simulink model "TSR_Scenario_002_cs"  (R2014b)
settings: Solver=ode5  SolverMode=SingleTasking  StartTime=0.0  StopTime=inf  FixedStep=1/100  RelTol=1e-3
PreLoadFcn:
  | mbxruntime.callbacks.PreLoadFcn(bdroot);
  | check_NUTS_defined;
  | 
  | assignin('base',['model_closed_' bdroot],false);
  | 
  | addpath('../includes_TSR/includes_TSR');
  | 
  | switch version('-release')
  | case {'2010a', '2010b', '2011a'}
  | addpath('../includes_TSR/ML2010b');
  | otherwise
  | addpath('../includes_TSR/ML2011b');
  | end
PostLoadFcn:
  | mbxruntime.callbacks.PostLoadFcn(bdroot);
InitFcn:
  | mbxruntime.callbacks.InitFcn(bdroot);;
  | 
  | addpath('..\includes_TSR');
StartFcn:
  | mbxruntime.callbacks.StartFcn(bdroot);
StopFcn:
  | mbxruntime.callbacks.StopFcn(bdroot);
model workspace: external: MAT-File .\TSR_Scenario_002_cs_hws.mat (data not in the file)
undefined symbols (not defined in the file or in its folder): InitImageOutputDir, mbxruntime, OrientationPitch, OrientationRoll, PositionX, PositionY, PositionZ, tabledata, warningInitialVelocity, x0
undefined symbols (not defined in the file): SteeringColumn, SteeringWheel, TSR_Scenario_002_cs_003e47b1b59594b6, TSR_Scenario_002_cs_023e87a31011dc74, TSR_Scenario_002_cs_048cb8409c90d9c6, TSR_Scenario_002_cs_106a0284aafa53e6, TSR_Scenario_002_cs_195b368d22a7f172, TSR_Scenario_002_cs_1e339fa5d680f213, TSR_Scenario_002_cs_26196a9fb104f950, TSR_Scenario_002_cs_261a709f6f453598, TSR_Scenario_002_cs_2ac3337370d0049d, TSR_Scenario_002_cs_2dc51e6a68b01b00, TSR_Scenario_002_cs_3460ff54d38ab2e2, TSR_Scenario_002_cs_42ea7d6e56bd6005, TSR_Scenario_002_cs_4dd419d6d2b56fc2, TSR_Scenario_002_cs_5316a21de09dff2f, TSR_Scenario_002_cs_538caacf3455966d, TSR_Scenario_002_cs_5b2cfdbcfc80811f, TSR_Scenario_002_cs_5ce0eafbb7a2dce7, TSR_Scenario_002_cs_62cdbf45c6f8824a, TSR_Scenario_002_cs_6bebc368eedff0bc, TSR_Scenario_002_cs_6d26481da4ed7e29, TSR_Scenario_002_cs_70c7e369ce6550e0, TSR_Scenario_002_cs_7a63051a1f311451, TSR_Scenario_002_cs_7d7dc8405f613c6d, TSR_Scenario_002_cs_7f65e296173485e8, TSR_Scenario_002_cs_87183cf6ff7bb4b6, TSR_Scenario_002_cs_8921b0da7ab80865, TSR_Scenario_002_cs_9495ce3a76763d1f, TSR_Scenario_002_cs_a679806a2fdc8099, TSR_Scenario_002_cs_Actros_1860_1_Path_pathUniqueID, TSR_Scenario_002_cs_Actros_2541_1_Path_pathUniqueID, TSR_Scenario_002_cs_Actros_2541_3_Path_pathUniqueID, TSR_Scenario_002_cs_Actros_2541_4_Path_pathUniqueID, TSR_Scenario_002_cs_adf24c93a9de8a4e, TSR_Scenario_002_cs_Audi_A8_1_Dynamics_Simple_initialPitch, TSR_Scenario_002_cs_Audi_A8_1_Dynamics_Simple_initialRoll, TSR_Scenario_002_cs_Audi_A8_1_Dynamics_Simple_initialX, TSR_Scenario_002_cs_Audi_A8_1_Dynamics_Simple_initialY, TSR_Scenario_002_cs_Audi_A8_1_Dynamics_Simple_initialYaw, TSR_Scenario_002_cs_Audi_A8_1_Dynamics_Simple_initialZ, TSR_Scenario_002_cs_b136c6ccb55f77db, TSR_Scenario_002_cs_ba4f809714c282b7, TSR_Scenario_002_cs_BMW_X5_1_Path_pathUniqueID, TSR_Scenario_002_cs_BMW_X5_1_SpeedProfile_speedProfileUniqueID, TSR_Scenario_002_cs_BMW_X5_2_Path_pathUniqueID, TSR_Scenario_002_cs_BMW_X5_2_SpeedProfile_speedProfileUniqueID, TSR_Scenario_002_cs_Citroen_C3_1_Path_pathUniqueID, TSR_Scenario_002_cs_Citroen_C3_2_Path_pathUniqueID, TSR_Scenario_002_cs_d8f275339b7082cf, TSR_Scenario_002_cs_Daf_95_1_Path_pathUniqueID, TSR_Scenario_002_cs_Daf_95_1_SpeedProfile_speedProfileUniqueID, TSR_Scenario_002_cs_dc019741510ce2f2, TSR_Scenario_002_cs_fdbc8aabe460b27c, TSR_Scenario_002_cs_Fiat_Bravo_1_Path_pathUniqueID, TSR_Scenario_002_cs_Ford_Fiesta_1_Path_pathUniqueID, TSR_Scenario_002_cs_Honda_Pan_European_1_Path_pathUniqueID, TSR_Scenario_002_cs_Mazda_RX8_1_Path_pathUniqueID, TSR_Scenario_002_cs_Nissan_Cabstar_1_Path_pathUniqueID, TSR_Scenario_002_cs_Nissan_Cabstar_2_Path_pathUniqueID ... (+9)
libraries: simulink_extras x82, simulink x23, PreScanSimulinkLibrary x11
(part 11 of 39)

== system TSR_Scenario_002_cs/HighwayOverhang_28 ==
  note: Resources
      |
      | 1: InformationSign\MatrixSign_GreenArrow.png: MatrixSign GreenArrow
      | 2: InformationSign\Empty.jpeg: Empty
      | 3: InformationSign\SEARCH_Logo.png: SEARCH Logo
      | 4: InformationSign\z274-50_black_full.png: z274-50 black full
      | 5: InformationSign\z274-51_black_full.png: z274-51 black full
      | 6: InformationSign\z274-52_black_full.png: z274-52 black full
      | 7: InformationSign\z274-53_black_full.png: z274-53 black full
      | 8: InformationSign\z274-54_black_full.png: z274-54 black full
      | 9: InformationSign\z274-55_black_full.png: z274-55 black full
      | 10: InformationSign\z274-56_black_full.png: z274-56 black full
      | 11: InformationSign\z274-57_black_full.png: z274-57 black full
      | 12: InformationSign\z274-58_black_full.png: z274-58 black full
      | 13: InformationSign\z274-59_black_full.png: z274-59 black full
      | 14: InformationSign\z274-60_black_full.png: z274-60 black full
      | 15: InformationSign\z274-61_black_full.png: z274-61 black full
      | 16: InformationSign\z274-62_black_full.png: z274-62 black full
      | 17: InformationSign\z274-63_black_full.png: z274-63 black full
  Ground_{1..4} (4 alike) : Ground
  VISUMatrixSignLights_Mux : Subsystem  Tag=mux/VisuMatrixSignLights  mask(PreScan User Interface: VisuMatrixSignLights){}
      mask help:
      | The VisuMatrixSignLights block provides a way to switch the lights on the matrix sign board on or off
      |
      | For more information, please click Help.
      mask Help: eval('openHelp(732)')
  VISUMatrixSign_Mux : Subsystem  Tag=mux/MatrixSign_v2  mask(PreScan User Interface: VisuMatrixSign){}
      mask help:
      | The VisuMatrixSign block provides a way to adapt the texture of the plates connected to an overhang, based on Resource IDs of the texture files.
      |
      | For more information, please click Help.
      settings: DeleteFcn=PreScanBlockDeleteFcn;
      mask Help: eval('openHelp(733)')
  VISUMatrixSign_HighwayOverhang_28 : Outport  Tag=outport/VisuMatrixSign  SampleTime=1/100
  VISUMatrixSignLights_HighwayOverhang_28 : Outport  Tag=outport/VisuMatrixSignLights  Port=2  SampleTime=1/100
  wires:
  VISUMatrixSign_Mux/1(MatrixSigns) -> VISUMatrixSign_HighwayOverhang_28/1
  VISUMatrixSignLights_Mux/1(VISUMatrixSignLights_HighwayOverhang_28) -> VISUMatrixSignLights_HighwayOverhang_28/1
  Ground_1/1 -> VISUMatrixSignLights_Mux/1(MatrixSign_41)
  Ground_2/1 -> VISUMatrixSignLights_Mux/2(MatrixSign_42)
  Ground_3/1 -> VISUMatrixSign_Mux/1(MatrixSign_41)
  Ground_4/1 -> VISUMatrixSign_Mux/2(MatrixSign_42)

== system TSR_Scenario_002_cs/HighwayOverhang_3 ==
  note: Resources
      |
      | 1: InformationSign\MatrixSign_GreenArrow.png: MatrixSign GreenArrow
      | 2: InformationSign\Empty.jpeg: Empty
      | 3: InformationSign\SEARCH_Logo.png: SEARCH Logo
      | 4: InformationSign\z274-50_black_full.png: z274-50 black full
      | 5: InformationSign\z274-51_black_full.png: z274-51 black full
      | 6: InformationSign\z274-52_black_full.png: z274-52 black full
      | 7: InformationSign\z274-53_black_full.png: z274-53 black full
      | 8: InformationSign\z274-54_black_full.png: z274-54 black full
      | 9: InformationSign\z274-55_black_full.png: z274-55 black full
      | 10: InformationSign\z274-56_black_full.png: z274-56 black full
      | 11: InformationSign\z274-57_black_full.png: z274-57 black full
      | 12: InformationSign\z274-58_black_full.png: z274-58 black full
      | 13: InformationSign\z274-59_black_full.png: z274-59 black full
      | 14: InformationSign\z274-60_black_full.png: z274-60 black full
      | 15: InformationSign\z274-61_black_full.png: z274-61 black full
      | 16: InformationSign\z274-62_black_full.png: z274-62 black full
      | 17: InformationSign\z274-63_black_full.png: z274-63 black full
  Ground_{1..4} (4 alike) : Ground
  VISUMatrixSignLights_Mux : Subsystem  Tag=mux/VisuMatrixSignLights  mask(PreScan User Interface: VisuMatrixSignLights){}
      mask help:
      | The VisuMatrixSignLights block provides a way to switch the lights on the matrix sign board on or off
      |
      | For more information, please click Help.
      mask Help: eval('openHelp(732)')
  VISUMatrixSign_Mux : Subsystem  Tag=mux/MatrixSign_v2  mask(PreScan User Interface: VisuMatrixSign){}
      mask help:
      | The VisuMatrixSign block provides a way to adapt the texture of the plates connected to an overhang, based on Resource IDs of the texture files.
      |
      | For more information, please click Help.
      settings: DeleteFcn=PreScanBlockDeleteFcn;
      mask Help: eval('openHelp(733)')
  VISUMatrixSign_HighwayOverhang_3 : Outport  Tag=outport/VisuMatrixSign  SampleTime=1/100
  VISUMatrixSignLights_HighwayOverhang_3 : Outport  Tag=outport/VisuMatrixSignLights  Port=2  SampleTime=1/100
  wires:
  VISUMatrixSign_Mux/1(MatrixSigns) -> VISUMatrixSign_HighwayOverhang_3/1
  VISUMatrixSignLights_Mux/1(VISUMatrixSignLights_HighwayOverhang_3) -> VISUMatrixSignLights_HighwayOverhang_3/1
  Ground_1/1 -> VISUMatrixSignLights_Mux/1(MatrixSign_12)
  Ground_2/1 -> VISUMatrixSignLights_Mux/2(MatrixSign_50)
  Ground_3/1 -> VISUMatrixSign_Mux/1(MatrixSign_12)
  Ground_4/1 -> VISUMatrixSign_Mux/2(MatrixSign_50)

== system TSR_Scenario_002_cs/HighwayOverhang_4 ==
  note: Resources
      |
      | 1: InformationSign\MatrixSign_GreenArrow.png: MatrixSign GreenArrow
      | 2: InformationSign\Empty.jpeg: Empty
      | 3: InformationSign\SEARCH_Logo.png: SEARCH Logo
      | 4: InformationSign\z274-50_black_full.png: z274-50 black full
      | 5: InformationSign\z274-51_black_full.png: z274-51 black full
      | 6: InformationSign\z274-52_black_full.png: z274-52 black full
      | 7: InformationSign\z274-53_black_full.png: z274-53 black full
      | 8: InformationSign\z274-54_black_full.png: z274-54 black full
      | 9: InformationSign\z274-55_black_full.png: z274-55 black full
      | 10: InformationSign\z274-56_black_full.png: z274-56 black full
      | 11: InformationSign\z274-57_black_full.png: z274-57 black full
      | 12: InformationSign\z274-58_black_full.png: z274-58 black full
      | 13: InformationSign\z274-59_black_full.png: z274-59 black full
      | 14: InformationSign\z274-60_black_full.png: z274-60 black full
      | 15: InformationSign\z274-61_black_full.png: z274-61 black full
      | 16: InformationSign\z274-62_black_full.png: z274-62 black full
      | 17: InformationSign\z274-63_black_full.png: z274-63 black full
  Ground_{1..4} (4 alike) : Ground
  VISUMatrixSignLights_Mux : Subsystem  Tag=mux/VisuMatrixSignLights  mask(PreScan User Interface: VisuMatrixSignLights){}
      mask help:
      | The VisuMatrixSignLights block provides a way to switch the lights on the matrix sign board on or off
      |
      | For more information, please click Help.
      mask Help: eval('openHelp(732)')
  VISUMatrixSign_Mux : Subsystem  Tag=mux/MatrixSign_v2  mask(PreScan User Interface: VisuMatrixSign){}
      mask help:
      | The VisuMatrixSign block provides a way to adapt the texture of the plates connected to an overhang, based on Resource IDs of the texture files.
      |
      | For more information, please click Help.
      settings: DeleteFcn=PreScanBlockDeleteFcn;
      mask Help: eval('openHelp(733)')
  VISUMatrixSign_HighwayOverhang_4 : Outport  Tag=outport/VisuMatrixSign  SampleTime=1/100
  VISUMatrixSignLights_HighwayOverhang_4 : Outport  Tag=outport/VisuMatrixSignLights  Port=2  SampleTime=1/100
  wires:
  VISUMatrixSign_Mux/1(MatrixSigns) -> VISUMatrixSign_HighwayOverhang_4/1
  VISUMatrixSignLights_Mux/1(VISUMatrixSignLights_HighwayOverhang_4) -> VISUMatrixSignLights_HighwayOverhang_4/1
  Ground_1/1 -> VISUMatrixSignLights_Mux/1(MatrixSign_23)
  Ground_2/1 -> VISUMatrixSignLights_Mux/2(MatrixSign_24)
  Ground_3/1 -> VISUMatrixSign_Mux/1(MatrixSign_23)
  Ground_4/1 -> VISUMatrixSign_Mux/2(MatrixSign_24)

== system TSR_Scenario_002_cs/HighwayOverhang_5 ==
  note: Resources
      |
      | 1: InformationSign\MatrixSign_GreenArrow.png: MatrixSign GreenArrow
      | 2: InformationSign\Empty.jpeg: Empty
      | 3: InformationSign\SEARCH_Logo.png: SEARCH Logo
      | 4: InformationSign\z274-50_black_full.png: z274-50 black full
      | 5: InformationSign\z274-51_black_full.png: z274-51 black full
      | 6: InformationSign\z274-52_black_full.png: z274-52 black full
      | 7: InformationSign\z274-53_black_full.png: z274-53 black full
      | 8: InformationSign\z274-54_black_full.png: z274-54 black full
      | 9: InformationSign\z274-55_black_full.png: z274-55 black full
      | 10: InformationSign\z274-56_black_full.png: z274-56 black full
      | 11: InformationSign\z274-57_black_full.png: z274-57 black full
      | 12: InformationSign\z274-58_black_full.png: z274-58 black full
      | 13: InformationSign\z274-59_black_full.png: z274-59 black full
      | 14: InformationSign\z274-60_black_full.png: z274-60 black full
      | 15: InformationSign\z274-61_black_full.png: z274-61 black full
      | 16: InformationSign\z274-62_black_full.png: z274-62 black full
      | 17: InformationSign\z274-63_black_full.png: z274-63 black full
  Ground_{1..4} (4 alike) : Ground
  VISUMatrixSignLights_Mux : Subsystem  Tag=mux/VisuMatrixSignLights  mask(PreScan User Interface: VisuMatrixSignLights){}
      mask help:
      | The VisuMatrixSignLights block provides a way to switch the lights on the matrix sign board on or off
      |
      | For more information, please click Help.
      mask Help: eval('openHelp(732)')
  VISUMatrixSign_Mux : Subsystem  Tag=mux/MatrixSign_v2  mask(PreScan User Interface: VisuMatrixSign){}
      mask help:
      | The VisuMatrixSign block provides a way to adapt the texture of the plates connected to an overhang, based on Resource IDs of the texture files.
      |
      | For more information, please click Help.
      settings: DeleteFcn=PreScanBlockDeleteFcn;
      mask Help: eval('openHelp(733)')
  VISUMatrixSign_HighwayOverhang_5 : Outport  Tag=outport/VisuMatrixSign  SampleTime=1/100
  VISUMatrixSignLights_HighwayOverhang_5 : Outport  Tag=outport/VisuMatrixSignLights  Port=2  SampleTime=1/100
  wires:
  VISUMatrixSign_Mux/1(MatrixSigns) -> VISUMatrixSign_HighwayOverhang_5/1
  VISUMatrixSignLights_Mux/1(VISUMatrixSignLights_HighwayOverhang_5) -> VISUMatrixSignLights_HighwayOverhang_5/1
  Ground_1/1 -> VISUMatrixSignLights_Mux/1(MatrixSign_48)
  Ground_2/1 -> VISUMatrixSignLights_Mux/2(MatrixSign_8)
  Ground_3/1 -> VISUMatrixSign_Mux/1(MatrixSign_8)
  Ground_4/1 -> VISUMatrixSign_Mux/2(MatrixSign_48)

== system TSR_Scenario_002_cs/HighwayOverhang_6 ==
  note: Resources
      |
      | 1: InformationSign\MatrixSign_GreenArrow.png: MatrixSign GreenArrow
      | 2: InformationSign\Empty.jpeg: Empty
      | 3: InformationSign\SEARCH_Logo.png: SEARCH Logo
      | 4: InformationSign\z274-50_black_full.png: z274-50 black full
      | 5: InformationSign\z274-51_black_full.png: z274-51 black full
      | 6: InformationSign\z274-52_black_full.png: z274-52 black full
      | 7: InformationSign\z274-53_black_full.png: z274-53 black full
      | 8: InformationSign\z274-54_black_full.png: z274-54 black full
      | 9: InformationSign\z274-55_black_full.png: z274-55 black full
      | 10: InformationSign\z274-56_black_full.png: z274-56 black full
      | 11: InformationSign\z274-57_black_full.png: z274-57 black full
      | 12: InformationSign\z274-58_black_full.png: z274-58 black full
      | 13: InformationSign\z274-59_black_full.png: z274-59 black full
      | 14: InformationSign\z274-60_black_full.png: z274-60 black full
      | 15: InformationSign\z274-61_black_full.png: z274-61 black full
      | 16: InformationSign\z274-62_black_full.png: z274-62 black full
      | 17: InformationSign\z274-63_black_full.png: z274-63 black full
  Ground_{1..4} (4 alike) : Ground
  VISUMatrixSignLights_Mux : Subsystem  Tag=mux/VisuMatrixSignLights  mask(PreScan User Interface: VisuMatrixSignLights){}
      mask help:
      | The VisuMatrixSignLights block provides a way to switch the lights on the matrix sign board on or off
      |
      | For more information, please click Help.
      mask Help: eval('openHelp(732)')
  VISUMatrixSign_Mux : Subsystem  Tag=mux/MatrixSign_v2  mask(PreScan User Interface: VisuMatrixSign){}
      mask help:
      | The VisuMatrixSign block provides a way to adapt the texture of the plates connected to an overhang, based on Resource IDs of the texture files.
      |
      | For more information, please click Help.
      settings: DeleteFcn=PreScanBlockDeleteFcn;
      mask Help: eval('openHelp(733)')
  VISUMatrixSign_HighwayOverhang_6 : Outport  Tag=outport/VisuMatrixSign  SampleTime=1/100
  VISUMatrixSignLights_HighwayOverhang_6 : Outport  Tag=outport/VisuMatrixSignLights  Port=2  SampleTime=1/100
  wires:
  VISUMatrixSign_Mux/1(MatrixSigns) -> VISUMatrixSign_HighwayOverhang_6/1
  VISUMatrixSignLights_Mux/1(VISUMatrixSignLights_HighwayOverhang_6) -> VISUMatrixSignLights_HighwayOverhang_6/1
  Ground_1/1 -> VISUMatrixSignLights_Mux/1(MatrixSign_19)
  Ground_2/1 -> VISUMatrixSignLights_Mux/2(MatrixSign_20)
  Ground_3/1 -> VISUMatrixSign_Mux/1(MatrixSign_19)
  Ground_4/1 -> VISUMatrixSign_Mux/2(MatrixSign_20)

== system TSR_Scenario_002_cs/HighwayOverhang_7 ==
  note: Resources
      |
      | 1: InformationSign\MatrixSign_GreenArrow.png: MatrixSign GreenArrow
      | 2: InformationSign\Empty.jpeg: Empty
      | 3: InformationSign\SEARCH_Logo.png: SEARCH Logo
      | 4: InformationSign\z274-50_black_full.png: z274-50 black full
      | 5: InformationSign\z274-51_black_full.png: z274-51 black full
      | 6: InformationSign\z274-52_black_full.png: z274-52 black full
      | 7: InformationSign\z274-53_black_full.png: z274-53 black full
      | 8: InformationSign\z274-54_black_full.png: z274-54 black full
      | 9: InformationSign\z274-55_black_full.png: z274-55 black full
      | 10: InformationSign\z274-56_black_full.png: z274-56 black full
      | 11: InformationSign\z274-57_black_full.png: z274-57 black full
      | 12: InformationSign\z274-58_black_full.png: z274-58 black full
      | 13: InformationSign\z274-59_black_full.png: z274-59 black full
      | 14: InformationSign\z274-60_black_full.png: z274-60 black full
      | 15: InformationSign\z274-61_black_full.png: z274-61 black full
      | 16: InformationSign\z274-62_black_full.png: z274-62 black full
      | 17: InformationSign\z274-63_black_full.png: z274-63 black full
  Ground_{1..4} (4 alike) : Ground
  VISUMatrixSignLights_Mux : Subsystem  Tag=mux/VisuMatrixSignLights  mask(PreScan User Interface: VisuMatrixSignLights){}
      mask help:
      | The VisuMatrixSignLights block provides a way to switch the lights on the matrix sign board on or off
      |
      | For more information, please click Help.
      mask Help: eval('openHelp(732)')
  VISUMatrixSign_Mux : Subsystem  Tag=mux/MatrixSign_v2  mask(PreScan User Interface: VisuMatrixSign){}
      mask help:
      | The VisuMatrixSign block provides a way to adapt the texture of the plates connected to an overhang, based on Resource IDs of the texture files.
      |
      | For more information, please click Help.
      settings: DeleteFcn=PreScanBlockDeleteFcn;
      mask Help: eval('openHelp(733)')
  VISUMatrixSign_HighwayOverhang_7 : Outport  Tag=outport/VisuMatrixSign  SampleTime=1/100
  VISUMatrixSignLights_HighwayOverhang_7 : Outport  Tag=outport/VisuMatrixSignLights  Port=2  SampleTime=1/100
  wires:
  VISUMatrixSign_Mux/1(MatrixSigns) -> VISUMatrixSign_HighwayOverhang_7/1
  VISUMatrixSignLights_Mux/1(VISUMatrixSignLights_HighwayOverhang_7) -> VISUMatrixSignLights_HighwayOverhang_7/1
  Ground_1/1 -> VISUMatrixSignLights_Mux/1(MatrixSign_4)
  Ground_2/1 -> VISUMatrixSignLights_Mux/2(MatrixSign_45)
  Ground_3/1 -> VISUMatrixSign_Mux/1(MatrixSign_4)
  Ground_4/1 -> VISUMatrixSign_Mux/2(MatrixSign_45)

== system TSR_Scenario_002_cs/HighwayOverhang_8 ==
  note: Resources
      |
      | 1: InformationSign\MatrixSign_GreenArrow.png: MatrixSign GreenArrow
      | 2: InformationSign\Empty.jpeg: Empty
      | 3: InformationSign\SEARCH_Logo.png: SEARCH Logo
      | 4: InformationSign\z274-50_black_full.png: z274-50 black full
      | 5: InformationSign\z274-51_black_full.png: z274-51 black full
      | 6: InformationSign\z274-52_black_full.png: z274-52 black full
      | 7: InformationSign\z274-53_black_full.png: z274-53 black full
      | 8: InformationSign\z274-54_black_full.png: z274-54 black full
      | 9: InformationSign\z274-55_black_full.png: z274-55 black full
      | 10: InformationSign\z274-56_black_full.png: z274-56 black full
      | 11: InformationSign\z274-57_black_full.png: z274-57 black full
      | 12: InformationSign\z274-58_black_full.png: z274-58 black full
      | 13: InformationSign\z274-59_black_full.png: z274-59 black full
      | 14: InformationSign\z274-60_black_full.png: z274-60 black full
      | 15: InformationSign\z274-61_black_full.png: z274-61 black full
      | 16: InformationSign\z274-62_black_full.png: z274-62 black full
      | 17: InformationSign\z274-63_black_full.png: z274-63 black full
  Ground_{1..4} (4 alike) : Ground
  VISUMatrixSignLights_Mux : Subsystem  Tag=mux/VisuMatrixSignLights  mask(PreScan User Interface: VisuMatrixSignLights){}
      mask help:
      | The VisuMatrixSignLights block provides a way to switch the lights on the matrix sign board on or off
      |
      | For more information, please click Help.
      mask Help: eval('openHelp(732)')
  VISUMatrixSign_Mux : Subsystem  Tag=mux/MatrixSign_v2  mask(PreScan User Interface: VisuMatrixSign){}
      mask help:
      | The VisuMatrixSign block provides a way to adapt the texture of the plates connected to an overhang, based on Resource IDs of the texture files.
      |
      | For more information, please click Help.
      settings: DeleteFcn=PreScanBlockDeleteFcn;
      mask Help: eval('openHelp(733)')
  VISUMatrixSign_HighwayOverhang_8 : Outport  Tag=outport/VisuMatrixSign  SampleTime=1/100
  VISUMatrixSignLights_HighwayOverhang_8 : Outport  Tag=outport/VisuMatrixSignLights  Port=2  SampleTime=1/100
  wires:
  VISUMatrixSign_Mux/1(MatrixSigns) -> VISUMatrixSign_HighwayOverhang_8/1
  VISUMatrixSignLights_Mux/1(VISUMatrixSignLights_HighwayOverhang_8) -> VISUMatrixSignLights_HighwayOverhang_8/1
  Ground_1/1 -> VISUMatrixSignLights_Mux/1(MatrixSign_15)
  Ground_2/1 -> VISUMatrixSignLights_Mux/2(MatrixSign_16)
  Ground_3/1 -> VISUMatrixSign_Mux/1(MatrixSign_15)
  Ground_4/1 -> VISUMatrixSign_Mux/2(MatrixSign_16)

== system TSR_Scenario_002_cs/HighwayOverhang_9 ==
  note: Resources
      |
      | 1: InformationSign\MatrixSign_GreenArrow.png: MatrixSign GreenArrow
      | 2: InformationSign\Empty.jpeg: Empty
      | 3: InformationSign\SEARCH_Logo.png: SEARCH Logo
      | 4: InformationSign\z274-50_black_full.png: z274-50 black full
      | 5: InformationSign\z274-51_black_full.png: z274-51 black full
      | 6: InformationSign\z274-52_black_full.png: z274-52 black full
      | 7: InformationSign\z274-53_black_full.png: z274-53 black full
      | 8: InformationSign\z274-54_black_full.png: z274-54 black full
      | 9: InformationSign\z274-55_black_full.png: z274-55 black full
      | 10: InformationSign\z274-56_black_full.png: z274-56 black full
      | 11: InformationSign\z274-57_black_full.png: z274-57 black full
      | 12: InformationSign\z274-58_black_full.png: z274-58 black full
      | 13: InformationSign\z274-59_black_full.png: z274-59 black full
      | 14: InformationSign\z274-60_black_full.png: z274-60 black full
      | 15: InformationSign\z274-61_black_full.png: z274-61 black full
      | 16: InformationSign\z274-62_black_full.png: z274-62 black full
      | 17: InformationSign\z274-63_black_full.png: z274-63 black full
  Ground_{1..4} (4 alike) : Ground
  VISUMatrixSignLights_Mux : Subsystem  Tag=mux/VisuMatrixSignLights  mask(PreScan User Interface: VisuMatrixSignLights){}
      mask help:
      | The VisuMatrixSignLights block provides a way to switch the lights on the matrix sign board on or off
      |
      | For more information, please click Help.
      mask Help: eval('openHelp(732)')
  VISUMatrixSign_Mux : Subsystem  Tag=mux/MatrixSign_v2  mask(PreScan User Interface: VisuMatrixSign){}
      mask help:
      | The VisuMatrixSign block provides a way to adapt the texture of the plates connected to an overhang, based on Resource IDs of the texture files.
      |
      | For more information, please click Help.
      settings: DeleteFcn=PreScanBlockDeleteFcn;
      mask Help: eval('openHelp(733)')
  VISUMatrixSign_HighwayOverhang_9 : Outport  Tag=outport/VisuMatrixSign  SampleTime=1/100
  VISUMatrixSignLights_HighwayOverhang_9 : Outport  Tag=outport/VisuMatrixSignLights  Port=2  SampleTime=1/100
  wires:
  VISUMatrixSign_Mux/1(MatrixSigns) -> VISUMatrixSign_HighwayOverhang_9/1
  VISUMatrixSignLights_Mux/1(VISUMatrixSignLights_HighwayOverhang_9) -> VISUMatrixSignLights_HighwayOverhang_9/1
  Ground_1/1 -> VISUMatrixSignLights_Mux/1(MatrixSign_47)
  Ground_2/1 -> VISUMatrixSignLights_Mux/2(MatrixSign_6)
  Ground_3/1 -> VISUMatrixSign_Mux/1(MatrixSign_6)
  Ground_4/1 -> VISUMatrixSign_Mux/2(MatrixSign_47)

== system TSR_Scenario_002_cs/Honda_Pan_European_1 ==
  SELF_Honda_Pan_European_1 : Inport  Tag=inport/SelfPort  OutDataTypeStr=Bus: PRESCAN_SELFSENSORDATA  PortDimensions=1  SampleTime=1/100  BusOutputAsStruct=on
  Path : S-Function  Tag=Path  LoadFcn=load('PrescanMotionData.mat')  FunctionName=sfun_Path  Parameters=uniqueID, pathUniqueID, timestep  EnableBusSupport=off  mask(Path){uniqueID=1163, pathUniqueID=TSR_Scenario_002_cs_Honda_Pan_European_1_Path_pathUniqueID, timestep=1/100}
      mask prompts: uniqueID "Object Unique ID"; pathUniqueID "Path Unique ID"; timestep "MATLAB timestep:"
      mask help:
      | The path block outputs the position along a given trajectory.
      |
      | For more information, please click Help.
      mask Help: eval('openHelp(312)')
      mask Display: image(imread('Path.png'))
  SELF_Demux : Subsystem  Tag=demux/SelfPort  mask(PreScan Demux Block:){}
      mask help:
      | The SELF port shows (state) information of the actor itself. The outputs are position in the experiment's axis system and the GPS coordinates, and the object's absolute velocity and compass heading.
      |
      | For more information, please click Help.
      settings: DeleteFcn=PreScanBlockDeleteFcn;
      mask Help: eval('openHelp(462)')
      mask Display:
      | port_label('output',1,'x [m]')
      | port_label('output',2,'y [m]')
      | port_label('output',3,'z [m]','texmode','on')
      | port_label('output',4,'Rotx [deg]','texmode','on')
      | port_label('output',5,'Roty [deg]','texmode','on')
      | port_label('output',6,'Rotz [deg]','texmode','on')
      | port_label('output',7,'GPS lat [deg]','texmode','on')
      | port_label('output',8,'GPS long [deg]','texmode','on')
      | port_label('output',9,'GPS alt [m]','texmode','on')
      | port_label('output',10,'Velocity [m/s]')
      | port_label('output',11,'Heading [deg]')
      | port_label('output',12,'Yaw rate [deg/s]')
  STATE_Honda_Pan_European_1_rc : RateTransition  Tag=mux_rc/StatePort  OutPortSampleTimeOpt=Inherit
  SpeedProfile : S-Function  Tag=SpeedProfile  LoadFcn=load('PrescanMotionData.mat')  FunctionName=sfun_SpeedProfile  Parameters=speedProfileUniqueID, timestep  EnableBusSupport=off  mask(SpeedProfile){speedProfileUniqueID=TSR_Scenario_002_cs_adf24c93a9de8a4e, timestep=1/100}
      mask prompts: speedProfileUniqueID "Speed Profile Unique ID"; timestep "MATLAB timestep:"
      mask help:
      | The speed profile block outputs the travelled distance, velocities and acceleration along a given path.
      |
      | For more information, please click Help.
      mask Help: eval('openHelp(312)')
      mask Display: image(imread('SpeedProfile.png'))
  Terminator_{1..12} (12 alike) : Terminator
  STATE_Honda_Pan_European_1_bus : Outport  Tag=outport/StatePort  OutDataTypeStr=Bus: PRESCAN_STATEACTUATORDATA  PortDimensions=1  SampleTime=1/100
  wires:
  STATE_Honda_Pan_European_1_rc/1 -> STATE_Honda_Pan_European_1_bus/1
  SpeedProfile/1 -> Path/1
  Path/1 -> STATE_Honda_Pan_European_1_rc/1
  SELF_Honda_Pan_European_1/1 -> SELF_Demux/1(SELF)
  SELF_Demux/1(x [m]) -> Terminator_1/1
  SELF_Demux/2(y [m]) -> Terminator_2/1
  SELF_Demux/3(z [m]) -> Terminator_3/1
  SELF_Demux/4(rotx [deg]) -> Terminator_4/1
  SELF_Demux/5(roty [deg]) -> Terminator_5/1
  SELF_Demux/6(rotz [deg]) -> Terminator_6/1
  SELF_Demux/7(GPS lat [deg]) -> Terminator_7/1
  SELF_Demux/8(GPS long [deg]) -> Terminator_8/1
  SELF_Demux/9(GPS alt [m]) -> Terminator_9/1
  SELF_Demux/10(velocity [m/s]) -> Terminator_10/1
  SELF_Demux/11(heading [deg]) -> Terminator_11/1
  SELF_Demux/12(yaw rate [deg/s]) -> Terminator_12/1

== system TSR_Scenario_002_cs/Male_RegularAni_1 ==
  SELF_Male_RegularAni_1 : Inport  Tag=inport/SelfPort  OutDataTypeStr=Bus: PRESCAN_SELFSENSORDATA  PortDimensions=1  SampleTime=1/100  BusOutputAsStruct=on
  Animation : Subsystem  Tag=RunningHumanAnimation  mask(Prescan Conversion Block: Running Human Animation){MWS=1.95, WalkingScale=1.0, RunningScale=0.22, TimeStep=1/100}
      mask prompts: MWS "Maximum Walking Speed [m/s], above which the animation will switch to running mode."; WalkingScale "Walking mode scaling factor to sync the animation frames to the displacement."; RunningScale "Running mode scaling factor to sync the animation frames to the displacement."; TimeStep "Auto-Assigned: Upload Period [s]"
      mask help: The Running Human Animation block converts the State signal of a human into signals to properly control the animation.
      mask Help: eval('openHelp(239)');
      mask Display: image(imread('HumanAnimated.jpg'))
  ColorRegion_Lower_Body_color : Constant  Tag=VisuLightConst  Value=[0 0 255]
  ColorRegion_Shoes_color : Constant  Tag=VisuLightConst  Value=[0 0 0]
  ColorRegion_Upper_Body_color : Constant  Tag=VisuLightConst  Value=[165 42 42]
  Dynamics_Empty : Subsystem  Tag=Dynamics_Empty
      mask Help: eval('openHelp(202)')
      mask Display: port_label('output', 1, 'State');text(0,0,' Empty\n')
  SELF_Demux : Subsystem  Tag=demux/SelfPort  mask(PreScan Demux Block:){}
      mask help:
      | The SELF port shows (state) information of the actor itself. The outputs are position in the experiment's axis system and the GPS coordinates, and the object's absolute velocity and compass heading.
      |
      | For more information, please click Help.
      settings: DeleteFcn=PreScanBlockDeleteFcn;
      mask Help: eval('openHelp(462)')
      mask Display:
      | port_label('output',1,'x [m]')
      | port_label('output',2,'y [m]')
      | port_label('output',3,'z [m]','texmode','on')
      | port_label('output',4,'Rotx [deg]','texmode','on')
      | port_label('output',5,'Roty [deg]','texmode','on')
      | port_label('output',6,'Rotz [deg]','texmode','on')
      | port_label('output',7,'GPS lat [deg]','texmode','on')
      | port_label('output',8,'GPS long [deg]','texmode','on')
      | port_label('output',9,'GPS alt [m]','texmode','on')
      | port_label('output',10,'Velocity [m/s]')
      | port_label('output',11,'Heading [deg]')
      | port_label('output',12,'Yaw rate [deg/s]')
  STATE_Male_RegularAni_1_rc : RateTransition  Tag=mux_rc/StatePort  OutPortSampleTimeOpt=Inherit
  Terminator_{1..12} (12 alike) : Terminator
  VISUColorRegion_Lower_Body_Mux : Subsystem  Tag=mux/MuxColorRegion  LoadFcn=load PrescanColorData  mask(PreScan User Interface: VisuTextureColor){}
      mask help:
      | The VisuTextureColor block provides a way to adapt the color of a vehicle.
      |
      | For more information, please click Help.
      settings: DeleteFcn=PreScanBlockDeleteFcn;
      mask Help: eval('openHelp(230)')
  VISUColorRegion_Shoes_Mux : Subsystem  Tag=mux/MuxColorRegion  LoadFcn=load PrescanColorData  mask(PreScan User Interface: VisuTextureColor){}
      mask help:
      | The VisuTextureColor block provides a way to adapt the color of a vehicle.
      |
      | For more information, please click Help.
      settings: DeleteFcn=PreScanBlockDeleteFcn;
      mask Help: eval('openHelp(230)')
  VISUColorRegion_Upper_Body_Mux : Subsystem  Tag=mux/MuxColorRegion  LoadFcn=load PrescanColorData  mask(PreScan User Interface: VisuTextureColor){}
      mask help:
      | The VisuTextureColor block provides a way to adapt the color of a vehicle.
      |
      | For more information, please click Help.
      settings: DeleteFcn=PreScanBlockDeleteFcn;
      mask Help: eval('openHelp(230)')
  STATE_Male_RegularAni_1_bus : Outport  Tag=outport/StatePort  OutDataTypeStr=Bus: PRESCAN_STATEACTUATORDATA  PortDimensions=1  SampleTime=1/100
  ANIM_Male_RegularAni_1 : Outport  Tag=outport/AnimationOutport  Port=2  OutDataTypeStr=Bus: PRESCAN_ANIMACTUATORDATA  PortDimensions=1  SampleTime=1/100
  VISUColorRegion_Upper_Body_Male_RegularAni_1 : Outport  Tag=outport/ColorRegion  Port=3  OutDataTypeStr=Bus: PRESCAN_COLOR_DATA  PortDimensions=1  SampleTime=1/100
  VISUColorRegion_Lower_Body_Male_RegularAni_1 : Outport  Tag=outport/ColorRegion  Port=4  OutDataTypeStr=Bus: PRESCAN_COLOR_DATA  PortDimensions=1  SampleTime=1/100
  VISUColorRegion_Shoes_Male_RegularAni_1 : Outport  Tag=outport/ColorRegion  Port=5  OutDataTypeStr=Bus: PRESCAN_COLOR_DATA  PortDimensions=1  SampleTime=1/100
  wires:
  Dynamics_Empty/1(State) -> Animation/1(In1), STATE_Male_RegularAni_1_rc/1
  STATE_Male_RegularAni_1_rc/1 -> STATE_Male_RegularAni_1_bus/1
  Animation/1(Out1) -> ANIM_Male_RegularAni_1/1
  SELF_Male_RegularAni_1/1 -> SELF_Demux/1(SELF)
  VISUColorRegion_Upper_Body_Mux/1(ColorRegion) -> VISUColorRegion_Upper_Body_Male_RegularAni_1/1
  ColorRegion_Upper_Body_color/1 -> VISUColorRegion_Upper_Body_Mux/1(RGB [-,-,-])
  VISUColorRegion_Lower_Body_Mux/1(ColorRegion) -> VISUColorRegion_Lower_Body_Male_RegularAni_1/1
  ColorRegion_Lower_Body_color/1 -> VISUColorRegion_Lower_Body_Mux/1(RGB [-,-,-])
  VISUColorRegion_Shoes_Mux/1(ColorRegion) -> VISUColorRegion_Shoes_Male_RegularAni_1/1
  ColorRegion_Shoes_color/1 -> VISUColorRegion_Shoes_Mux/1(RGB [-,-,-])
  SELF_Demux/1(x [m]) -> Terminator_1/1
  SELF_Demux/2(y [m]) -> Terminator_2/1
  SELF_Demux/3(z [m]) -> Terminator_3/1
  SELF_Demux/4(rotx [deg]) -> Terminator_4/1
  SELF_Demux/5(roty [deg]) -> Terminator_5/1
  SELF_Demux/6(rotz [deg]) -> Terminator_6/1
  SELF_Demux/7(GPS lat [deg]) -> Terminator_7/1
  SELF_Demux/8(GPS long [deg]) -> Terminator_8/1
  SELF_Demux/9(GPS alt [m]) -> Terminator_9/1
  SELF_Demux/10(velocity [m/s]) -> Terminator_10/1
  SELF_Demux/11(heading [deg]) -> Terminator_11/1
  SELF_Demux/12(yaw rate [deg/s]) -> Terminator_12/1

== system TSR_Scenario_002_cs/Mazda_RX8_1 ==
  SELF_Mazda_RX8_1 : Inport  Tag=inport/SelfPort  OutDataTypeStr=Bus: PRESCAN_SELFSENSORDATA  PortDimensions=1  SampleTime=1/100  BusOutputAsStruct=on
  Path : S-Function  Tag=Path  LoadFcn=load('PrescanMotionData.mat')  FunctionName=sfun_Path  Parameters=uniqueID, pathUniqueID, timestep  EnableBusSupport=off  mask(Path){uniqueID=1069, pathUniqueID=TSR_Scenario_002_cs_Mazda_RX8_1_Path_pathUniqueID, timestep=1/100}
      mask prompts: uniqueID "Object Unique ID"; pathUniqueID "Path Unique ID"; timestep "MATLAB timestep:"
      mask help:
      | The path block outputs the position along a given trajectory.
      |
      | For more information, please click Help.
      mask Help: eval('openHelp(312)')
      mask Display: image(imread('Path.png'))
  SELF_Demux : Subsystem  Tag=demux/SelfPort  mask(PreScan Demux Block:){}
      mask help:
      | The SELF port shows (state) information of the actor itself. The outputs are position in the experiment's axis system and the GPS coordinates, and the object's absolute velocity and compass heading.
      |
      | For more information, please click Help.
      settings: DeleteFcn=PreScanBlockDeleteFcn;
      mask Help: eval('openHelp(462)')
      mask Display:
      | port_label('output',1,'x [m]')
      | port_label('output',2,'y [m]')
      | port_label('output',3,'z [m]','texmode','on')
      | port_label('output',4,'Rotx [deg]','texmode','on')
      | port_label('output',5,'Roty [deg]','texmode','on')
      | port_label('output',6,'Rotz [deg]','texmode','on')
      | port_label('output',7,'GPS lat [deg]','texmode','on')
      | port_label('output',8,'GPS long [deg]','texmode','on')
      | port_label('output',9,'GPS alt [m]','texmode','on')
      | port_label('output',10,'Velocity [m/s]')
      | port_label('output',11,'Heading [deg]')
      | port_label('output',12,'Yaw rate [deg/s]')
  STATE_Mazda_RX8_1_rc : RateTransition  Tag=mux_rc/StatePort  OutPortSampleTimeOpt=Inherit
  SpeedProfile : S-Function  Tag=SpeedProfile  LoadFcn=load('PrescanMotionData.mat')  FunctionName=sfun_SpeedProfile  Parameters=speedProfileUniqueID, timestep  EnableBusSupport=off  mask(SpeedProfile){speedProfileUniqueID=TSR_Scenario_002_cs_2dc51e6a68b01b00, timestep=1/100}
      mask prompts: speedProfileUniqueID "Speed Profile Unique ID"; timestep "MATLAB timestep:"
      mask help:
      | The speed profile block outputs the travelled distance, velocities and acceleration along a given path.
      |
      | For more information, please click Help.
      mask Help: eval('openHelp(312)')
      mask Display: image(imread('SpeedProfile.png'))
  Terminator_{1..12} (12 alike) : Terminator
  STATE_Mazda_RX8_1_bus : Outport  Tag=outport/StatePort  OutDataTypeStr=Bus: PRESCAN_STATEACTUATORDATA  PortDimensions=1  SampleTime=1/100
  wires:
  STATE_Mazda_RX8_1_rc/1 -> STATE_Mazda_RX8_1_bus/1
  SpeedProfile/1 -> Path/1
  Path/1 -> STATE_Mazda_RX8_1_rc/1
  SELF_Mazda_RX8_1/1 -> SELF_Demux/1(SELF)
  SELF_Demux/1(x [m]) -> Terminator_1/1
  SELF_Demux/2(y [m]) -> Terminator_2/1
  SELF_Demux/3(z [m]) -> Terminator_3/1
  SELF_Demux/4(rotx [deg]) -> Terminator_4/1
  SELF_Demux/5(roty [deg]) -> Terminator_5/1
  SELF_Demux/6(rotz [deg]) -> Terminator_6/1
  SELF_Demux/7(GPS lat [deg]) -> Terminator_7/1
  SELF_Demux/8(GPS long [deg]) -> Terminator_8/1
  SELF_Demux/9(GPS alt [m]) -> Terminator_9/1
  SELF_Demux/10(velocity [m/s]) -> Terminator_10/1
  SELF_Demux/11(heading [deg]) -> Terminator_11/1
  SELF_Demux/12(yaw rate [deg/s]) -> Terminator_12/1
